simulink model "VOOstateflow"  (R2022a)
settings: Solver=FixedStepAuto  StartTime=0.0  StopTime=10.0  FixedStep=1e-3  RelTol=1e-3  EnableMultiTasking=on
libraries: frdmk64flib x1
settings Model: ExtModeTrigDuration=5  Creator=sabri  LastModifiedBy=sabri
settings SolverCC: AlgebraicLoopSolver=TrustRegion
settings OptimizationCC: EnhancedBackFolding=on  PassReuseOutputArgsAs=Individual arguments  ZeroExternalMemoryAtStartup=off  ZeroInternalMemoryAtStartup=off  MaxStackSize=64  OptimizeBlockOrder=speed  DifferentSizesBufferReuse=on  OptimizationCustomize=off  EfficientTunableParamExpr=on
settings DebuggingCC: ParameterTunabilityLossMsg=error  UnconnectedInputMsg=warning  UnconnectedOutputMsg=warning  UnconnectedLineMsg=warning  SFMachineParentedDataDiag=warning
settings HardwareCC: ProdBitPerPointer=32  ProdBitPerSizeT=32  ProdBitPerPtrDiffT=32  ProdLargestAtomicInteger=Long  ProdLargestAtomicFloat=Double  ProdWordSize=32  ProdHWDeviceType=ARM Compatible->ARM Cortex
settings SFSimCC: MATLABDynamicMemAlloc=off
settings RTWCC: SystemTargetFile=ert.tlc  HardwareBoard=NXP FRDM-K64F  TLCOptions="-aInlineSetEventsForThisBaseRateFcn=TLC_FALSE -aSuppressMultiTaskScheduler=TLC_FALSE  -aRateBasedStepFcn=0"  TemplateMakefile=ert_default_tmf  Toolchain=GNU Tools for ARM Embedded Processors
settings CodeAppCC: ForceParamTrailComments=on  IgnoreCustomStorageClasses=off  OperatorAnnotations=on  SimulinkDataObjDesc=on  SFDataObjDesc=on  InsertBlockDesc=on

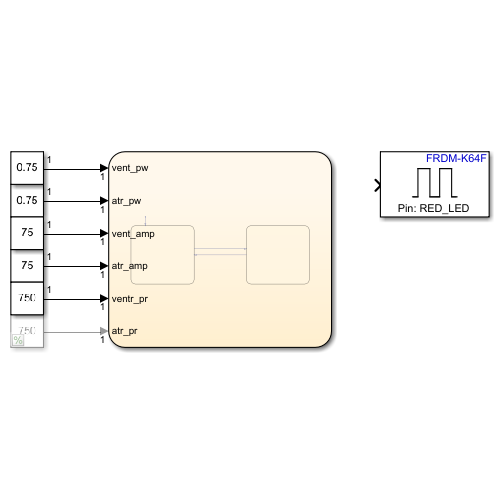
[thumbnail: Simulink's stored preview of the top-level diagram]
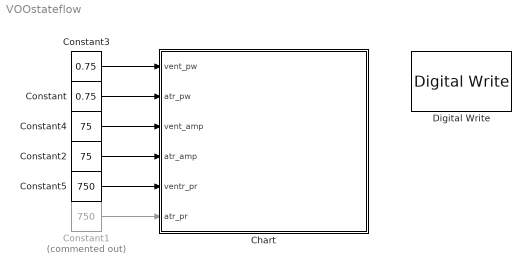
== system VOOstateflow ==
  Chart : Stateflow chart  TreatAsAtomicUnit=on
  Constant : Constant  Value=0.75
  Constant1 : Constant  Commented=on  Value=750
  Constant2 : Constant  Value=75
  Constant3 : Constant  Value=0.75
  Constant4 : Constant  Value=75
  Constant5 : Constant  Value=750
  Digital Write : frdmk64flib/Digital Write  Whichpin=RED_LED
  wires:
  Constant/1 -> Chart/2(atr_pw)
  Constant1/1 -> Chart/6(atr_pr)
  Constant2/1 -> Chart/4(atr_amp)
  Constant3/1 -> Chart/1(vent_pw)
  Constant4/1 -> Chart/3(vent_amp)
  Constant5/1 -> Chart/5(ventr_pr)

== stateflow chart VOOstateflow/Chart ==
  state Charging_Heart
    entry:
    PACE_CHARGE_CTRL = 0
    VENT_PACE_CTRL = 1
    ATR_PACE_CTRL = 0
    VENT_GND_CTRL = 0
    ATR_GND_CTRL = 0
    PACE_GND_CTRL = 1
    FRONTEND_CTRL = 0
    PACING_REF_PWM = vent_amp
  state Discharging_Heart
    entry:
    PACE_CHARGE_CTRL = 1
    VENT_PACE_CTRL = 0
    ATR_PACE_CTRL = 0
    VENT_GND_CTRL = 1
    ATR_GND_CTRL = 0
    PACE_GND_CTRL = 1
    FRONTEND_CTRL = 0
  (default) -> Charging_Heart
  Charging_Heart -> Discharging_Heart : [after(vent_pr - vent_pw, msec)]
  Discharging_Heart -> Charging_Heart : [after(vent_pw, msec)]
  data: vent_pw input; atr_pw input; vent_amp input; atr_amp input; ventr_pr input; atr_pr input
